simulink model "myFZPI"  (R2021a)
settings: Solver=ode15s  StartTime=0.0  StopTime=30  FixedStep=1  MaxStep=1  RelTol=1e-2  EnableMultiTasking=on
model workspace (MAT data in the model file):
  K = 5
  K1 = 5
  Kd = 12.5
  Ke = 2.5
  MaxError = 150
  Ts = 0.01
libraries: SignalEditorBlockLib x2, fuzblock x1
settings Model: SnapshotBufferSize=800  SnapshotInterval=1  EnablePacing=on  PacingRate=0.010000  Creator=harry  LastModifiedBy=harry
settings SolverCC: ConcurrentTasks=on  AlgebraicLoopSolver=TrustRegion  AutoInsertRateTranBlk=on
settings DataIOCC: ReturnWorkspaceOutputs=off
settings DebuggingCC: SFMachineParentedDataDiag=warning  ArithmeticOperatorsInVariantConditions=warning
settings SFSimCC: SimUseLocalCustomCode=off  CustomCodeUndefinedFunction=UseInterfaceOnly
settings RTWCC: RTWUseLocalCustomCode=off

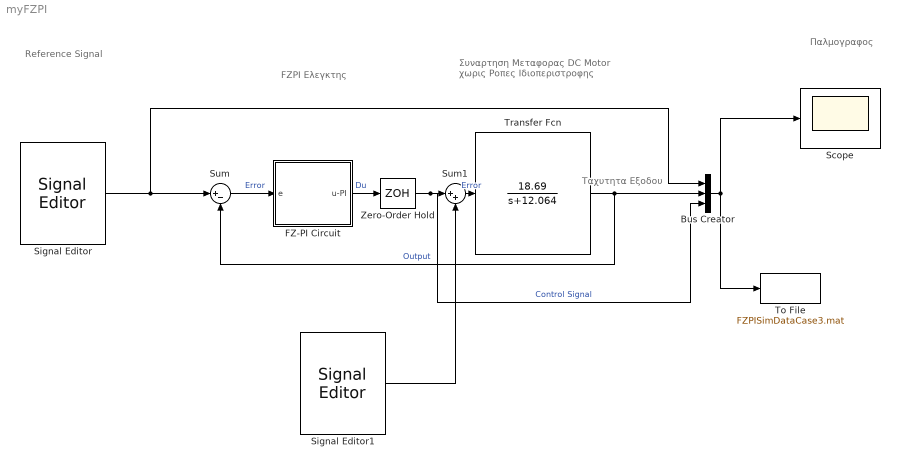
== system myFZPI ==
  note: Reference Signal
  note: FZPI Ελεγκτης
  note: Ταχυτητα Εξοδου
  note: Παλμογραφος
  note: Συναρτηση Μεταφορας DC Motor
      |  χωρις Ροπες Ιδιοπεριστροφης
  Bus Creator : BusCreator  Inputs=3
  FZ-PI Circuit : Subsystem
  Scope : Scope
  Signal Editor : SignalEditorBlockLib/Signal Editor  FileName=SignalCase3.mat  ActiveScenario=Scenario  ActiveSignal=input3  IsBus=off  OutputBusObjectStr=Bus: BusObject  SampleTime=0  Interpolate=off  ZeroCross=off  OutputAfterFinalValue=Setting to zero  Unit=inherit  PreserveSignalName=on
  Signal Editor1 : SignalEditorBlockLib/Signal Editor  FileName=DisturbSignalCase3.mat  ActiveScenario=Scenario  ActiveSignal=disturb3  IsBus=off  OutputBusObjectStr=Bus: BusObject  SampleTime=0  Interpolate=off  ZeroCross=off  OutputAfterFinalValue=Setting to zero  Unit=inherit  PreserveSignalName=on
  Sum : Sum  Inputs=|+-
  Sum1 : Sum  Inputs=|++
  To File : ToFile  Filename=FZPISimDataCase3.mat  MatrixName=FZPISimData  SaveFormat=Timeseries
  Transfer Fcn : TransferFcn  Description=DC Motor Transfer Function  Numerator=[18.69]  Denominator=[1 12.064]  ContinuousStateAttributes='RotationSpeed'
  Zero-Order Hold : ZeroOrderHold  SampleTime=0.01
  wires:
  Transfer Fcn/1 -> Bus Creator/2, Sum/2  "Output"
  Bus Creator/1 -> To File/1, Scope/1
  Sum/1 -> FZ-PI Circuit/1(e)  "Error"
  FZ-PI Circuit/1(u-PI) -> Zero-Order Hold/1  "Du"
  Zero-Order Hold/1 -> Bus Creator/3, Sum1/1  "Control Signal"
  Signal Editor/1 -> Bus Creator/1, Sum/1
  Sum1/1 -> Transfer Fcn/1  "Error"
  Signal Editor1/1 -> Sum1/2

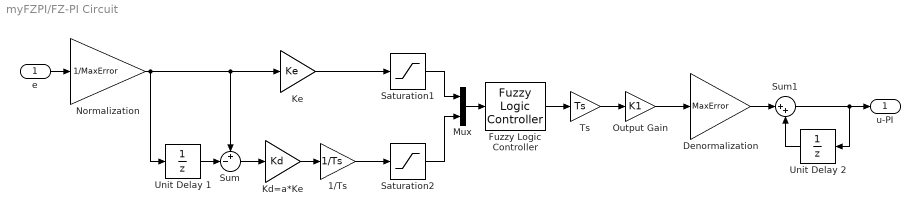
== system myFZPI/FZ-PI Circuit ==
  e : Inport
  1/Ts : Gain  Gain=1/Ts
  Denormalization : Gain  Gain=MaxError
  Fuzzy Logic Controller : fuzblock/Fuzzy Logic  Controller  FIS='FZPI.fis'  OutputSampleNumber=101  DataType=double  FuzzifiedInputs=off  RuleFiringStrengths=off  RuleOutputs=off  AggregatedOutputs=off  SimulateUsing=Interpreted execution  OutOfRangeInputValueMessage=warning  NoRuleFiredMessage=warning  EmptyOutputFuzzySetMessage=warning
  Kd=a*Ke : Gain  Gain=Kd
  Ke : Gain  Gain=Ke
  Mux : Mux  Inputs=2
  Normalization : Gain  Gain=1/MaxError
  Output Gain : Gain  Gain=K1
  "Saturation1 " : Saturate  UpperLimit=1  LowerLimit=-1
  Saturation2 : Saturate  UpperLimit=1  LowerLimit=-1
  Sum : Sum  Inputs=+-|
  Sum1 : Sum  Inputs=|++
  "Ts " : Gain  Gain=Ts
  Unit Delay 1 : UnitDelay  SampleTime=-1  HasFrameUpgradeWarning=on
  Unit Delay 2 : UnitDelay  SampleTime=-1  HasFrameUpgradeWarning=on
  u-PI : Outport  VectorParamsAs1DForOutWhenUnconnected=off
  wires:
  e/1 -> Normalization/1
  Mux/1 -> Fuzzy Logic Controller/1
  "Saturation1 "/1 -> Mux/1
  Normalization/1 -> Sum/1, Ke/1, Unit Delay 1/1
  Ke/1 -> "Saturation1 "/1
  Kd=a*Ke/1 -> 1/Ts/1
  1/Ts/1 -> Saturation2/1
  Saturation2/1 -> Mux/2
  Unit Delay 1/1 -> Sum/2
  Sum/1 -> Kd=a*Ke/1
  Sum1/1 -> u-PI/1, Unit Delay 2/1
  Unit Delay 2/1 -> Sum1/2
  Denormalization/1 -> Sum1/1
  Output Gain/1 -> Denormalization/1
  "Ts "/1 -> Output Gain/1
  Fuzzy Logic Controller/1 -> "Ts "/1
